simulink model "mmdlwks3"  (Simulink 6.3)
settings: Solver=FixedStepDiscrete  StartTime=0.0  StopTime=10.0  RelTol=1e-3
model workspace: external: MAT-File (data not in the file)
undefined symbols (not defined in the file or in its folder): k
CloseFcn:
  | rtwprivate ssgencode ModelCloseRequest prob1
settings Model: Creator=stoeppe  LastModifiedBy=mshakeri  ExtModeEnableOpenProtocolUploading=on  ExtModeOpenProtocolUploadingEqualLengthVectors=off  ExtModeAutoUpdateStatusClock=off  StrictBusMsg=ErrorLevel1
settings DataIOCC: SaveFormat=StructureWithTime  SignalLoggingName=sigsOut
settings OptimizationCC: InlineParams=on  OptimizeModelRefInitCode=on  LifeSpan=1
settings DebuggingCC: SigSpecEnsureSampleTime=on  SignalResolutionControl=UseLocalSettings  SolverPrmCheckMsg=none
settings HardwareCC: TargetUnknown=on
settings RTWCC: SystemTargetFile=ert.tlc  GenCodeOnly=on  TemplateMakefile=ert_default_tmf  GenerateReport=on  ProcessScript=ert_make_rtw_hook  IncludeHyperlinkInReport=on  LaunchReport=on
settings CodeAppCC: IgnoreCustomStorageClasses=off
settings ERTTargetCC: TargetFcnLib=ansi_tfl_tmw.mat  GenFloatMathFcnCalls=ANSI_C  GenerateSampleERTMain=on  InlinedParameterPlacement=NonHierarchical  ERTCustomFileTemplate=example_file_process.tlc  InitialValueSource=Model

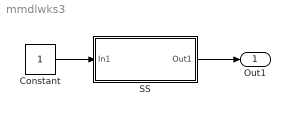
== system mmdlwks3 ==
  Constant : Constant  SampleTime=1
  SS : Subsystem  TreatAsAtomicUnit=on
  Out1 : Outport
  wires:
  Constant/1 -> SS/1(In1)
  SS/1(Out1) -> Out1/1

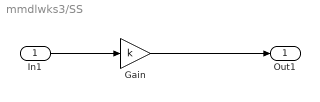
== system mmdlwks3/SS ==
  In1 : Inport  Port=1
  Gain : Gain  Gain=k
  Out1 : Outport
  wires:
  In1/1 -> Gain/1
  Gain/1 -> Out1/1
